simulink model "LAB02"  (R2023b)
settings: Solver=VariableStepAuto  StartTime=0.0  StopTime=0.2  RelTol=1e-3  AbsTol=1e-3
libraries: spsRMSLib x7, spsSeriesRLCBranchLib x3, spsACVoltageSourceLib x3, spsGroundLib x3, eePowerMeasurement x2, spsThreePhaseVIMeasurementLib x2, spsVoltageMeasurementLib x2, spsCurrentMeasurementLib x1, sps_lib x1
settings Model: Creator=sagar  LastModifiedBy=sagar
settings SolverCC: AutoScaleAbsTol=off  AlgebraicLoopSolver=TrustRegion  MaxZcPerStep=1
settings DebuggingCC: UnconnectedInputMsg=warning  UnconnectedOutputMsg=warning  UnconnectedLineMsg=warning  SymbolicDimsDataTypeCodeGenerationDiagnostic=none
settings ModelReferenceCC: EnableRefExpFcnMdlSchedulingChecks=on
settings SFSimCC: CustomCodeUndefinedFunction=UseInterfaceOnly
settings RTWCC: DLArmComputeVersion=19.05
settings SimscapeCC: SimscapeLogType=all  SimscapeLogSimulationStatistics=on  SimscapeLogDataHistory=10000

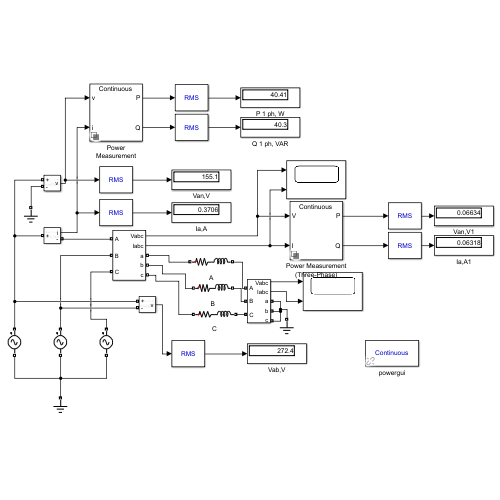
[thumbnail: Simulink's stored preview of the top-level diagram]
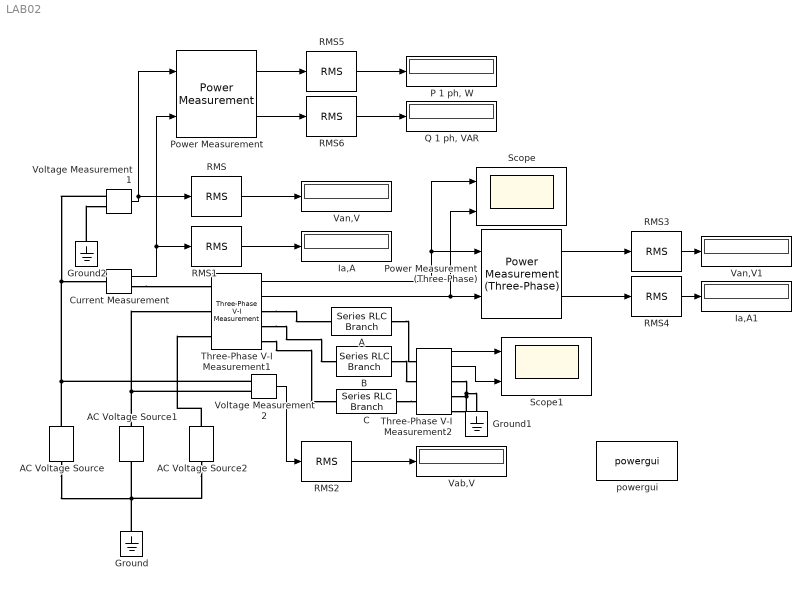
== system LAB02 ==
  A : spsSeriesRLCBranchLib/Series RLC Branch  LConnTagsString=__new0  RConnTagsString=__new0  BranchType=RL  Resistance=300  Inductance=0.9555  SetiL0=on  InitialCurrent=2  Capacitance=1e-6  Setx0=off  InitialVoltage=0  Measurements=None
  AC Voltage Source : spsACVoltageSourceLib/AC Voltage Source  Amplitude=220  Phase=0  Frequency=50  SampleTime=0  Measurements=None  BusType=swing  Pref=10e3  Qref=0  Qmin=-inf  Qmax=+inf
  AC Voltage Source1 : spsACVoltageSourceLib/AC Voltage Source  Amplitude=220  Phase=120  Frequency=50  SampleTime=0  Measurements=None  BusType=swing  Pref=10e3  Qref=0  Qmin=-inf  Qmax=+inf
  AC Voltage Source2 : spsACVoltageSourceLib/AC Voltage Source  Amplitude=220  Phase=240  Frequency=50  SampleTime=0  Measurements=None  BusType=swing  Pref=10e3  Qref=0  Qmin=-inf  Qmax=+inf
  B : spsSeriesRLCBranchLib/Series RLC Branch  LConnTagsString=__new0  RConnTagsString=__new0  BranchType=RL  Resistance=300  Inductance=0.9555  SetiL0=on  InitialCurrent=2  Capacitance=1e-6  Setx0=off  InitialVoltage=0  Measurements=None
  C : spsSeriesRLCBranchLib/Series RLC Branch  LConnTagsString=__new0  RConnTagsString=__new0  BranchType=RL  Resistance=300  Inductance=0.9555  SetiL0=on  InitialCurrent=2  Capacitance=1e-6  Setx0=off  InitialVoltage=0  Measurements=None
  Current Measurement : spsCurrentMeasurementLib/Current Measurement  PhasorSimulation=off  OutputType=Complex  PSBequivalent=0
  Ground : spsGroundLib/Ground  LConnTagsString=a
  Ground1 : spsGroundLib/Ground  LConnTagsString=a
  Ground2 : spsGroundLib/Ground  LConnTagsString=a
  Ia,A : Display
  Ia,A1 : Display
  "P 1 ph, W" : Display
  Power Measurement : eePowerMeasurement/Power Measurement  LabelModeActiveChoice=Continuous  F=50  K=[1]  Ts=0
  Power Measurement (Three-Phase) : eePowerMeasurement/Power Measurement (Three-Phase)  LabelModeActiveChoice=Continuous  F=50  K=[1]  Seq=Positive  Ts=0
  "Q 1 ph, VAR" : Display
  RMS{,1..6} (7 alike) : spsRMSLib/RMS  TrueRMS=on  Freq=50  RMSInit=120  Ts=0
  Scope : Scope  NumInputPorts=2
  Scope1 : Scope  NumInputPorts=2
  Three-Phase V-I Measurement1 : spsThreePhaseVIMeasurementLib/Three-Phase V-I Measurement  VoltageMeasurement=phase-to-ground  SetLabelV=off  LabelV=Vabc  Vpu=off  VpuLL=off  CurrentMeasurement=yes  SetLabelI=off  LabelI=Iabc  Ipu=off  Pbase=100e6  Vbase=500e3  OutputType=Complex  PhasorSimulation=off  PSBequivalent=0
  Three-Phase V-I Measurement2 : spsThreePhaseVIMeasurementLib/Three-Phase V-I Measurement  VoltageMeasurement=phase-to-ground  SetLabelV=off  LabelV=Vabc  Vpu=off  VpuLL=off  CurrentMeasurement=yes  SetLabelI=off  LabelI=Iabc  Ipu=off  Pbase=100e6  Vbase=500e3  OutputType=Complex  PhasorSimulation=off  PSBequivalent=0
  Vab,V : Display
  Van,V : Display
  Van,V1 : Display
  Voltage Measurement1 : spsVoltageMeasurementLib/Voltage Measurement  PhasorSimulation=off  OutputType=Complex  PSBequivalent=0
  Voltage Measurement2 : spsVoltageMeasurementLib/Voltage Measurement  PhasorSimulation=off  OutputType=Complex  PSBequivalent=0
  powergui : sps_lib/powergui  Priority=1  SimulationMode=Continuous  SampleTime=50e-6  frequency=50  Iterations=50  frequencyindice=50  Pbase=100e6  ErrMax=1e-4  UnitsV=kV  UnitsW=MW  buscounter=0  FunctionMessages=off  echomessages=off  EnableUseOfTLC=off  CurrentSourceSwitches=off  DisableSnubberDevices=off  DisableRonSwitches=off  DisableVfSwitches=off  DisplayEquations=off  AutomaticDiscreteSolvers=off  SolverType=Tustin/Backward Euler (TBE)  Interpol=off  ExternalGateDelay=off  methode=off  Ts=100  x0status=blocks  SPID=on  SwTol=0  HookPort=off  NonlinearTolerance=1e-4  nMaxIteration=100  ContinueOnMaxIteration=off  RestoreLinks=warning  ResistiveCurrentMeasurement=off  Frange=[0:2:500]  Ylog=off  Xlog=on  ShowGrid=off  save=off  variable=ZData  structure=0  ZoomFFT=off  StartTime=0.0  cycles=1  DisplayStyle=1  fundamental=60  FreqAxis=off  MaxFrequency=1000  frequencyindicesteady=1  RmsSteady=1  display=off
  wires:
  Voltage Measurement1/1 -> Power Measurement/1, RMS/1
  RMS/1 -> Van,V/1
  RMS1/1 -> Ia,A/1
  Current Measurement/1 -> Power Measurement/2, RMS1/1
  Power Measurement/1 -> RMS5/1
  Power Measurement/2 -> RMS6/1
  Three-Phase V-I Measurement1/1 -> Scope/1, Power Measurement (Three-Phase)/1
  Three-Phase V-I Measurement1/2 -> Scope/2, Power Measurement (Three-Phase)/2
  Voltage Measurement2/1 -> RMS2/1
  RMS2/1 -> Vab,V/1
  Three-Phase V-I Measurement2/1 -> Scope1/1
  Three-Phase V-I Measurement2/2 -> Scope1/2
  RMS4/1 -> Ia,A1/1
  RMS3/1 -> Van,V1/1
  Power Measurement (Three-Phase)/1 -> RMS3/1
  Power Measurement (Three-Phase)/2 -> RMS4/1
  RMS6/1 -> "Q 1 ph, VAR"/1
  RMS5/1 -> "P 1 ph, W"/1
  connections:
  AC Voltage Source/RConn1 -- Voltage Measurement2/LConn1 -- Voltage Measurement1/LConn1 -- Current Measurement/LConn1
  AC Voltage Source/LConn1 -- AC Voltage Source2/LConn1 -- Ground/LConn1 -- AC Voltage Source1/LConn1
  AC Voltage Source1/RConn1 -- Voltage Measurement2/LConn2 -- Three-Phase V-I Measurement1/LConn2
  Current Measurement/RConn1 -- Three-Phase V-I Measurement1/LConn1
  AC Voltage Source2/RConn1 -- Three-Phase V-I Measurement1/LConn3
  Three-Phase V-I Measurement1/RConn1 -- A/LConn1
  Three-Phase V-I Measurement1/RConn2 -- B/LConn1
  Three-Phase V-I Measurement1/RConn3 -- C/LConn1
  Ground2/LConn1 -- Voltage Measurement1/LConn2
  A/RConn1 -- Three-Phase V-I Measurement2/LConn1
  B/RConn1 -- Three-Phase V-I Measurement2/LConn2
  C/RConn1 -- Three-Phase V-I Measurement2/LConn3
  Three-Phase V-I Measurement2/RConn3 -- Three-Phase V-I Measurement2/RConn1 -- Ground1/LConn1 -- Three-Phase V-I Measurement2/RConn2
